simulink model "fixed_wing_model"  (R2021a)
settings: Solver=VariableStepAuto  StartTime=0.0  StopTime=20  RelTol=1e-3
settings Model: Creator=diogo  LastModifiedBy=Nunes
settings SolverCC: AlgebraicLoopSolver=TrustRegion
settings DebuggingCC: SFMachineParentedDataDiag=warning

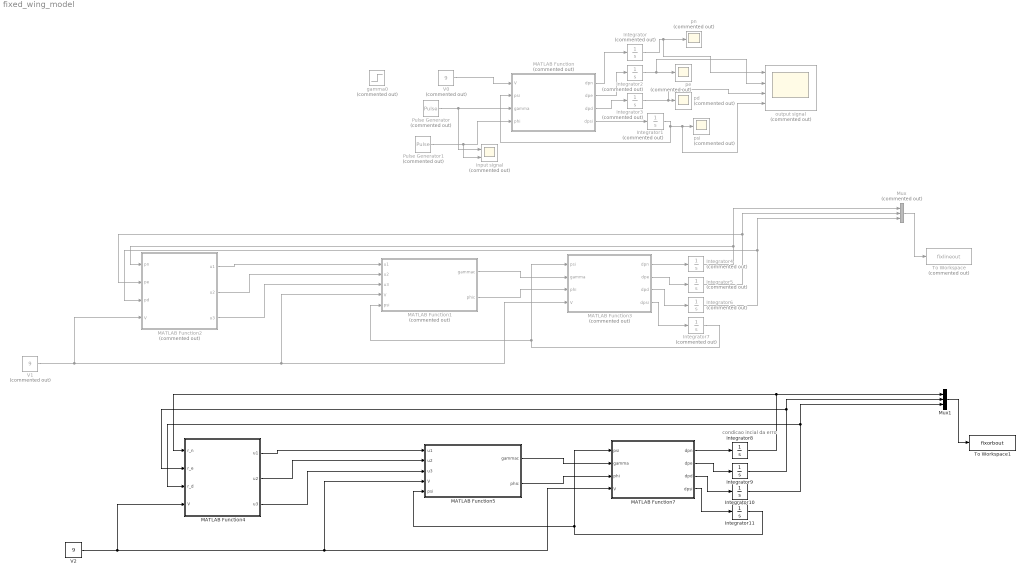
== system fixed_wing_model ==
  note: condicao incial da erro
  Integrator{,1..7} (8 alike) : Integrator  Commented=on
  Integrator10 : Integrator
  Integrator11 : Integrator
  Integrator8 : Integrator  InitialCondition=0.1
  Integrator9 : Integrator
  MATLAB Function : MATLAB Function  Commented=on  TreatAsAtomicUnit=on
  MATLAB Function1 : MATLAB Function  Commented=on  TreatAsAtomicUnit=on
  MATLAB Function2 : MATLAB Function  Commented=on  TreatAsAtomicUnit=on
  MATLAB Function3 : MATLAB Function  Commented=on  TreatAsAtomicUnit=on
  MATLAB Function4 : MATLAB Function  TreatAsAtomicUnit=on
  MATLAB Function5 : MATLAB Function  TreatAsAtomicUnit=on
  MATLAB Function7 : MATLAB Function  TreatAsAtomicUnit=on
  Mux : Mux  Commented=on  Inputs=3
  Mux1 : Mux  Inputs=3
  Pulse Generator : DiscretePulseGenerator  Commented=on  PulseType=Time based  Amplitude=0.087266  Period=20  PulseWidth=15  PhaseDelay=2
  Pulse Generator1 : DiscretePulseGenerator  Commented=on  PulseType=Time based  Amplitude=0.087266  Period=20  PulseWidth=15  PhaseDelay=13
  To Workspace : ToWorkspace  Commented=on  VariableName=fixlineout  SaveFormat=Timeseries  SampleTime=-1
  To Workspace1 : ToWorkspace  VariableName=fixorbout  SaveFormat=Timeseries  SampleTime=-1
  V0 : Constant  Commented=on  Value=9
  V1 : Constant  Commented=on  Value=9
  V2 : Constant  Value=9
  gamma0 : Step  Commented=on  Time=5  After=0.087266  SampleTime=0
  input signal : Scope  Commented=on  NumInputPorts=2
  output signal : Scope  Commented=on  NumInputPorts=4
  pd : Scope  Commented=on
  pe : Scope  Commented=on
  pn : Scope  Commented=on
  psi : Scope  Commented=on
  wires:
  MATLAB Function/1(dpn) -> Integrator/1
  MATLAB Function/4(dpsi) -> Integrator1/1
  Integrator/1 -> output signal/1, pn/1
  Integrator1/1 -> output signal/4, psi/1, MATLAB Function/2(psi)
  V0/1 -> MATLAB Function/1(V)
  Pulse Generator1/1 -> input signal/2, MATLAB Function/4(phi)
  MATLAB Function/2(dpe) -> Integrator2/1
  MATLAB Function/3(dpd) -> Integrator3/1
  Integrator2/1 -> output signal/2, pe/1
  Integrator3/1 -> output signal/3, pd/1
  Pulse Generator/1 -> input signal/1, MATLAB Function/3(gamma)
  MATLAB Function3/2(dpe) -> Integrator5/1
  MATLAB Function3/3(dpd) -> Integrator6/1
  MATLAB Function3/1(dpn) -> Integrator4/1
  MATLAB Function3/4(dpsi) -> Integrator7/1
  Integrator7/1 -> MATLAB Function1/5(psi), MATLAB Function3/1(psi)
  MATLAB Function1/2(phic) -> MATLAB Function3/3(phi)
  MATLAB Function1/1(gammac) -> MATLAB Function3/2(gamma)
  V1/1 -> MATLAB Function2/4(V), MATLAB Function1/4(V), MATLAB Function3/4(V)
  Integrator4/1 -> MATLAB Function2/1(pn), Mux/1
  Integrator5/1 -> MATLAB Function2/2(pe), Mux/2
  Integrator6/1 -> Mux/3, MATLAB Function2/3(pd)
  MATLAB Function2/1(u1) -> MATLAB Function1/1(u1)
  MATLAB Function2/2(u2) -> MATLAB Function1/2(u2)
  MATLAB Function2/3(u3) -> MATLAB Function1/3(u3)
  Mux/1 -> To Workspace/1
  MATLAB Function5/2(phic) -> MATLAB Function7/3(phi)
  Integrator9/1 -> MATLAB Function4/2(r_e), Mux1/2
  MATLAB Function7/1(dpn) -> Integrator8/1
  Integrator10/1 -> Mux1/3, MATLAB Function4/3(r_d)
  V2/1 -> MATLAB Function4/4(V), MATLAB Function5/4(V), MATLAB Function7/4(V)
  MATLAB Function7/4(dpsi) -> Integrator11/1
  MATLAB Function7/2(dpe) -> Integrator9/1
  Integrator11/1 -> MATLAB Function5/5(psi), MATLAB Function7/1(psi)
  Mux1/1 -> To Workspace1/1
  MATLAB Function5/1(gammac) -> MATLAB Function7/2(gamma)
  Integrator8/1 -> MATLAB Function4/1(r_n), Mux1/1
  MATLAB Function7/3(dpd) -> Integrator10/1
  MATLAB Function4/1(u1) -> MATLAB Function5/1(u1)
  MATLAB Function4/2(u2) -> MATLAB Function5/2(u2)
  MATLAB Function4/3(u3) -> MATLAB Function5/3(u3)

== matlab function fixed_wing_model/MATLAB Function1 ==
  data: u1 input; u2 input; u3 input; V input; psi input; gammac output; phic output
function [  gammac, phic] = path_following_controller(u1, u2, u3, V, psi)

%fazer isto como deve ser
gamma_limit = pi;
phi_limit = pi;
kphi = 1;

gammac = -sat(asin(u3/V), gamma_limit);

psid = atan2(u2,u1);

phic = sat(kphi*(psid- psi), phi_limit);

end

== matlab function fixed_wing_model/MATLAB Function ==
  data: V input; dpn output; dpe output; dpd output; psi input; gamma input; phi input; dpsi output
function [dpn, dpe, dpd,dpsi] = drone_model(V,psi,gamma,phi)
    
    %criar param para generalizar os valores
    
    %dp = [V*cos(psi)*cos(gamma); V*sin(psi)*cos(gamma); -V*sin(gamma)]
    
    dpn =V*cos(psi)*cos(gamma);
    dpe = V*sin(psi)*cos(gamma);
    dpd = -V*sin(gamma);
    dpsi =  (9.8/V)*tan(phi);
    
    
end

== matlab function fixed_wing_model/MATLAB Function2 ==
  data: pn input; u1 output; pe input; pd input; V input; u2 output; u3 output
function [u1, u2, u3] = straight_path_generator(pn, pe, pd, V)


%Variables

psi_l = 3*pi/4;  %desired heading angle
gamma_l = pi; %desired flight path angle

c_n = 1;    %path starting point
c_e = 1;
c_d = 1;

r_n = pn;    %position
r_e = pe;
r_d = pd;
r = [r_n; r_e; r_d];

cl = [c_n; c_e; c_d];
%point on the line (start position?)
ql = [cos(psi_l)*cos(gamma_l) ; sin(psi_l)*cos(gamma_l) ; -sin(gamma_l) ];
%direction of line




n_lon = [ -sin(psi_l) ; cos(psi_l) ; 0 ]; 

n_lat = cross(n_lon, ql);

k1 = 1;
k2 = 1;

u_line = k1*(n_lon*transpose(n_lon) +  n_lat*transpose(n_lat))*(r - cl) + k2*cross(n_lon,n_lat);

u = V*(u_line/norm(u_line));

u1 = u(1);
u2 = u(2);
u3 = u(3);


end

== matlab function fixed_wing_model/MATLAB Function3 ==
  data: psi input; gamma input; phi input; V input; dpn output; dpe output; dpd output; dpsi output
function [dpn, dpe, dpd,dpsi] = drone_model(psi,gamma,phi, V)
    
    %criar param para generalizar os valores
    
    %dp = [V*cos(psi)*cos(gamma); V*sin(psi)*cos(gamma); -V*sin(gamma)]
    
    dpn =V*cos(psi)*cos(gamma);
    dpe = V*sin(psi)*cos(gamma);
    dpd = -V*sin(gamma);
    dpsi =  (9.8/V)*tan(phi);
    
    
end

== matlab function fixed_wing_model/MATLAB Function4 ==
  data: r_n input; u1 output; r_e input; r_d input; V input; u2 output; u3 output
function [u1, u2, u3] = orbit_path_generator(r_n, r_e, r_d, V)


%Variables

 Rh = 30;
 lambda = 1;
 gamma_h = 0;%=15*pi/180;
 psi_h = 0;
 
k1 = 1;
k2 = 1;
 
c_n = 0;    %center of helix
c_e = 0;
c_d = 0;
ch = [c_n; c_e; c_d];

 %starting position

r0 = ch + [Rh*cos(psi_h) ; Rh*sin(psi_h) ; 0];

dalpha_cyl = transpose( [ 2*(r_n - c_n)/Rh ; 2*(r_e - c_e)/Rh ; 0 ] );

dalpha_pl = transpose( [ (tan(gamma_h)/lambda)*(-(r_e - c_e))/( (r_n - c_n)^2 + (r_e - c_e)^2 ) ; (tan(gamma_h)/lambda)*(r_n - c_e)/( (r_n - c_n)^2 + (r_e - c_e)^2 )  ; 1/Rh ] );


alpha_cyl = ( (r_n - c_n)/Rh )^2 + ( (r_e - c_e)/Rh )^2 -1;

alpha_pl = ( (r_d - c_d)/Rh )^2 + (tan(gamma_h)/lambda)*(atan( (r_e - c_e)/(r_n - c_n) ) - psi_h);

u_line = k1*(alpha_cyl*dalpha_cyl + alpha_pl*dalpha_pl) + lambda*k2*( (2/Rh)*transpose([ (r_e - c_e)/Rh ; -(r_n - c_n)/Rh ; lambda*tan(gamma_h) ]) );

u = V*(u_line/norm(u_line));


u1 = u(1);
u2 = u(2);
u3 = u(3);



end

== matlab function fixed_wing_model/MATLAB Function5 ==
  data: u1 input; u2 input; u3 input; V input; psi input; gammac output; phic output
function [  gammac, phic] = path_following_controller(u1, u2, u3, V, psi)

%fazer isto como deve ser
gamma_limit = pi;
phi_limit = pi;
kphi = 1;

gammac = -sat(asin(u3/V), gamma_limit);

psid = atan2(u2,u1);

phic = sat(kphi*(psid- psi), phi_limit);

end

== matlab function fixed_wing_model/MATLAB Function7 ==
  data: psi input; gamma input; phi input; V input; dpn output; dpe output; dpd output; dpsi output
function [dpn, dpe, dpd,dpsi] = drone_model(psi,gamma,phi, V)
    
    %criar param para generalizar os valores
    
    %dp = [V*cos(psi)*cos(gamma); V*sin(psi)*cos(gamma); -V*sin(gamma)]
    
    dpn =V*cos(psi)*cos(gamma);
    dpe = V*sin(psi)*cos(gamma);
    dpd = -V*sin(gamma);
    dpsi =  (9.8/V)*tan(phi);
    
    
end
